simulink model "motor"  (R2016a)
settings: Solver=VariableStepAuto  StartTime=0.0  StopTime=100  RelTol=1e-3
settings Model: Creator=Shahin  LastModifiedBy=Shahin

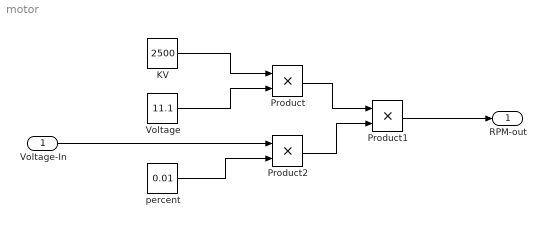
== system motor ==
  Voltage-In : Inport
  KV : Constant  Value=2500
  Product : Product
  Product1 : Product
  Product2 : Product
  Voltage : Constant  Value=11.1
  percent : Constant  Value=0.01
  RPM-out : Outport
  wires:
  KV/1 -> Product/1
  Voltage/1 -> Product/2
  Voltage-In/1 -> Product2/1
  percent/1 -> Product2/2
  Product/1 -> Product1/1
  Product2/1 -> Product1/2
  Product1/1 -> RPM-out/1
